simulink model "PI_CONTROLLER_Model_Ref"  (R2020b)
settings: Solver=VariableStepAuto  StartTime=0.0  StopTime=120  RelTol=1e-3
model mask{Ki=0.185, Kp=2.28}
PreLoadFcn:
  | vars
model workspace (MAT data in the model file):
  Ki = 0.185
  Kp = 2.28
values from neighbouring files (symbols this model uses):
  Ts = 0.01    [variables.m]
settings Model: DataDictionary=problem_3.sldd  ParameterArgumentNames=Ki,Kp  Creator=hp  LastModifiedBy=hp
settings DataIOCC: SaveOutput=off  SaveTime=off
settings DebuggingCC: ModelReferenceExtraNoncontSigs=none

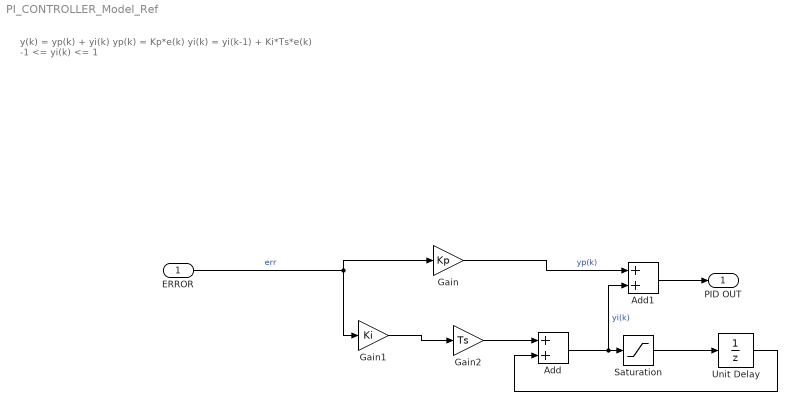
== system PI_CONTROLLER_Model_Ref ==
  note: y(k) = yp(k) + yi(k)
      |
      | yp(k) = Kp*e(k)
      |
      | yi(k) = yi(k-1) + Ki*Ts*e(k)
      |
      | -1 <= yi(k) <= 1
  ERROR : Inport  OutDataTypeStr=double  PortDimensions=1  SampleTime=0
  Add : Sum
  Add1 : Sum
  Gain : Gain  Gain=Kp
  Gain1 : Gain  Gain=Ki
  Gain2 : Gain  Gain=Ts
  Saturation : Saturate  UpperLimit=1  LowerLimit=-1
  Unit Delay : UnitDelay  SampleTime=-1  HasFrameUpgradeWarning=on
  PID OUT : Outport  OutDataTypeStr=double  PortDimensions=1  SampleTime=0
  wires:
  Add1/1 -> PID OUT/1
  Saturation/1 -> Unit Delay/1
  Gain2/1 -> Add/1
  Gain/1 -> Add1/1  "yp(k)"
  ERROR/1 -> Gain/1, Gain1/1  "err"
  Gain1/1 -> Gain2/1
  Unit Delay/1 -> Add/2
  Add/1 -> Saturation/1, Add1/2  "yi(k)"
